simulink model "AdaptiveModulation_HelmetAntenna"  (R2024b)
settings: Solver=FixedStepAuto  StartTime=0.0  StopTime=200  FixedStep=1  RelTol=1e-3
settings Model: Creator=ARYA MGC  LastModifiedBy=ARYA MGC

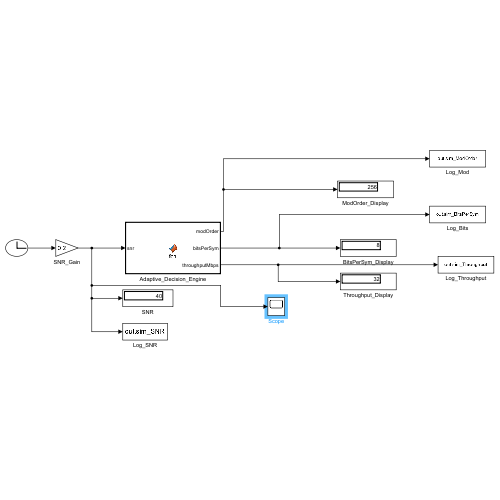
[thumbnail: Simulink's stored preview of the top-level diagram]
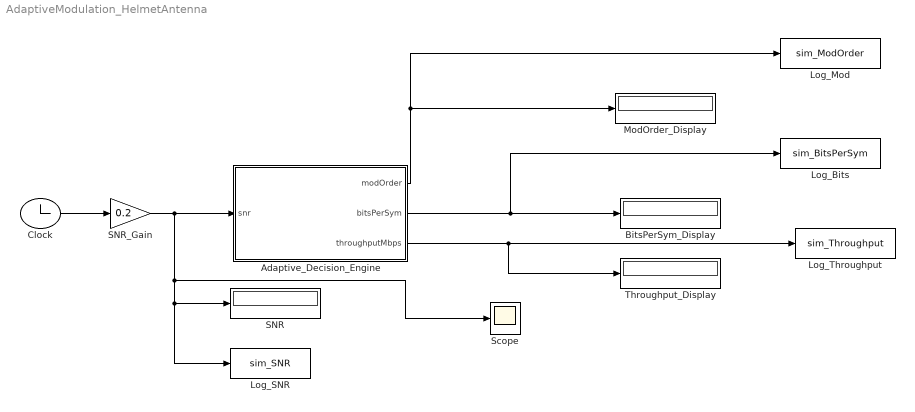
== system AdaptiveModulation_HelmetAntenna ==
  Adaptive_Decision_Engine : MATLAB Function  TreatAsAtomicUnit=on
  BitsPerSym_Display : Display
  Clock : Clock
  Log_Bits : ToWorkspace  VariableName=sim_BitsPerSym  SampleTime=-1
  Log_Mod : ToWorkspace  VariableName=sim_ModOrder  SampleTime=-1
  Log_SNR : ToWorkspace  VariableName=sim_SNR  SampleTime=-1
  Log_Throughput : ToWorkspace  VariableName=sim_Throughput  SampleTime=-1
  ModOrder_Display : Display
  SNR : Display
  SNR_Gain : Gain  Gain=0.2
  Scope : Scope
  Throughput_Display : Display
  wires:
  Clock/1 -> SNR_Gain/1
  SNR_Gain/1 -> Adaptive_Decision_Engine/1(snr), Scope/1, SNR/1, Log_SNR/1
  Adaptive_Decision_Engine/1(modOrder) -> ModOrder_Display/1, Log_Mod/1
  Adaptive_Decision_Engine/2(bitsPerSym) -> Log_Bits/1, BitsPerSym_Display/1
  Adaptive_Decision_Engine/3(throughputMbps) -> Throughput_Display/1, Log_Throughput/1

== matlab function AdaptiveModulation_HelmetAntenna/Adaptive_Decision_Engine ==
  data: snr input; modOrder output; bitsPerSym output; throughputMbps output
function [modOrder, bitsPerSym, throughputMbps] = fcn(snr)
BW = 4;  % Channel bandwidth (MHz)
if snr >= 26
    modOrder = 256; bitsPerSym = 8;  % 256-QAM
elseif snr >= 20
    modOrder = 64;  bitsPerSym = 6;  % 64-QAM
elseif snr >= 14
    modOrder = 16;  bitsPerSym = 4;  % 16-QAM
elseif snr >= 8
    modOrder = 4;   bitsPerSym = 2;  % QPSK
else
    modOrder = 2;   bitsPerSym = 1;  % BPSK
end
throughputMbps = bitsPerSym * BW;
